simulink model "CustomLidarSLAM"  (R2024a)
settings: Solver=VariableStepAuto  StartTime=0.0  StopTime=10  RelTol=1e-3
values from neighbouring files (symbols this model uses):
  refPosesT = [180 179.9129385 179.835485475 179.767633325 179.70937525 179.660705309 179.62161846 179.592110609 179.572178633 179.56182041 179.561034833 179.569821817 ... (300 elements, 300x1)]    [refPosesT.mat]
  refPosesX = [39.2750629723 38.6655653744 38.0559809852 37.4463199178 36.8365922852 36.2268082005 35.6169777769 35.0071111275 34.3972183654 33.7873096037 33.1773949554 32.5674845338 ... (300 elements, 300x1)]    [refPosesX.mat]
  refPosesY = [28.2732997481 28.27377135 28.2751181677 28.2772382193 28.2800295229 28.2833900965 28.2872179581 28.2914111258 28.2958676177 28.3004854519 28.3051626463 28.3097972191 ... (300 elements, 300x1)]    [refPosesY.mat]
undefined symbols (not defined in the file or in its folder): Sim3dSensor
libraries: sim3dphyssensorlib x1, sim3dlib x1, sim3dautolib x1
settings Model: Creator=The MathWorks, Inc.  LastModifiedBy=FilippoOttaviani
settings SolverCC: AlgebraicLoopSolver=TrustRegion
settings DebuggingCC: UnconnectedInputMsg=warning  UnconnectedOutputMsg=warning  UnconnectedLineMsg=warning  SymbolicDimsDataTypeCodeGenerationDiagnostic=none
settings ModelReferenceCC: EnableRefExpFcnMdlSchedulingChecks=on
settings RTWCC: GPUComputeCapability=3.5  DLArmComputeVersion=19.05

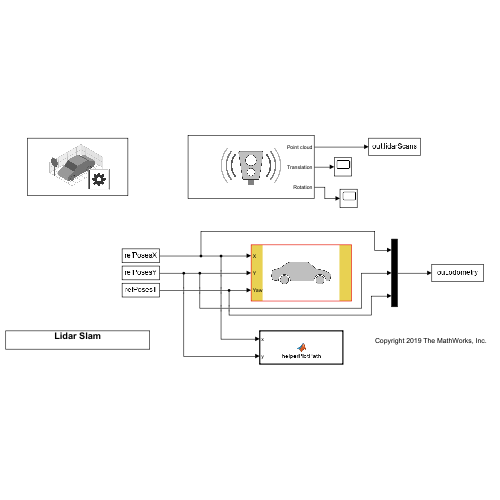
[thumbnail: Simulink's stored preview of the top-level diagram]
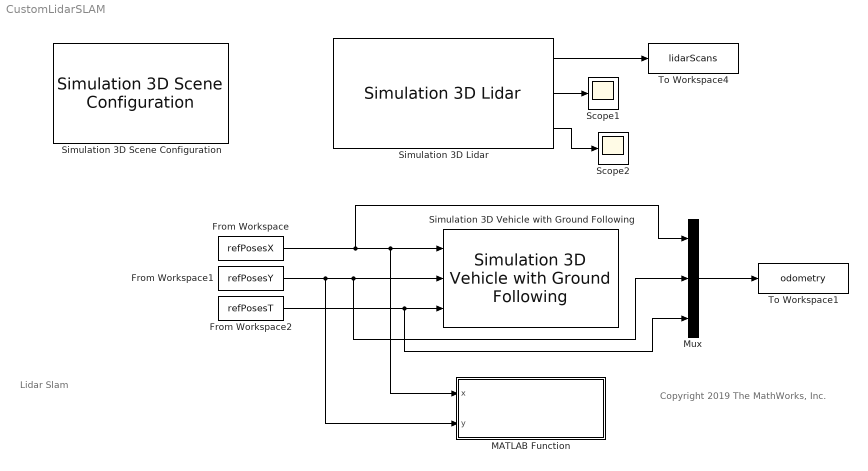
== system CustomLidarSLAM ==
  note: Copyright 2019 The MathWorks, Inc.
  note: Lidar Slam
  From Workspace : FromWorkspace  VariableName=refPosesX
  From Workspace1 : FromWorkspace  VariableName=refPosesY
  From Workspace2 : FromWorkspace  VariableName=refPosesT  Interpolate=off  OutputAfterFinalValue=Holding final value
  MATLAB Function : MATLAB Function  TreatAsAtomicUnit=on
      settings: ModelCloseFcn=|
      | % Find figure with name "Scene Display"
      | hFig = findobj('Type', 'figure', 'Name', 'Scene Display');
      | 
      | if ~isempty(hFig) && isvalid(hFig)
      |     close(hFig);
      | end
      | clear hFig;
  Mux : Mux  Inputs=3
  Scope1 : Scope
  Scope2 : Scope
  Simulation 3D Lidar : sim3dphyssensorlib/Simulation 3D Lidar  Priority=1  sensorTag=Sim3dSensor�  sensorId=1  sensorName=Sim3dSensor�  vehTagList={'Scene Origin';'SimulinkVehicle1'}  vehTag=SimulinkVehicle1  mountLoc=Roof center  offsetFlag=off  tmountOffset=[0, 0, 0]  rmountOffset=[0, 0, 0]  DetectionRange=30  RangeResolution=0.01  VerticalFOV=40  VerticalResolution=1.25  HorizontalFOV=360  HorizontalResolution=1  DistanceOutportEnabled=off  ReflectivityOutportEnabled=off  SemanticOutportEnabled=off  TransformOutportEnabled=on  SampleTime=-1  mountPoint=[-0.25 0 1.57000005245209]  mountOrientation=[0 0 0]  aMode=5  ID=1
      settings: LibrarySourceBlock=sl3dlib/Simulation 3D/Sensors/Simulation 3D Lidar
  Simulation 3D Scene Configuration : sim3dlib/Simulation 3D Scene Configuration  Priority=0  ProjectFormat=Default Scenes  SceneDesc=Large parking lot  ProjectName=C:\Program Files\MATLAB\R2024a\toolbox\shared\sim3d_projects\automotive_project_windows\UE\WindowsNoEditor\VehicleSimulation.exe  ScenePath=/Game/Maps/HwStrght  EnableOpenDRIVE=off  vehTagList={'Custom';'Scene Origin';'SimulinkVehicle1'}  vehTag=SimulinkVehicle1  FreeCameraInitialTranslation=[0, 0, 0]  FreeCameraDefaultInitialTranslation=[-6, 0, 2]  FreeCameraInitialRotation=[0, 0, 0]  FreeCameraDefaultInitialRotation=[0, -15, 0]  OpVisEn=off  Ts=1/60  EnableWindow=on  EnableRemoteAccess=off  EnableWeather=off  SunAzimuth=90  SunAltitude=40.0  EnableGeospatialSun=off  Latitude=0  Longitude=0  Date=2023-01-01  Time=10:30:00  GeoTimeZone=-5.0  SunDaylightSaving=off  wind=1  clouds=10  EnableVolumetricClouds=off  CloudCoverage=0  CloudAltitude=6  fog=0  rain=0  RaindropsEffect=off  SnowDensity=0  EnableGeospatial=off  UseTrueOrigin=off  OriginHeight=200  OriginLatitude=40.744652  OriginLongitude=-73.988864  MapStyle=Aerial  AdditionalAssetIDs=[]  UseAdvancedSunSky=off  SolarTime=11  TimeZone=-5  Day=21  Month=9  Year=2022  UseDaylightSavingTime=on  DSTStartDay=10  DSTStartMonth=3  DSTEndDay=3  DSTEndMonth=11  DSTSwitchHour=2  sensorTag=MainCamera2  sensorId=2  sensorName=MainCamera2  mountLoc=Origin  offsetFlag=off  tmountOffset=[0, 0, 0]  rmountOffset=[0, 0, 0]  HorizontalResolution=1280  VerticalResolution=720  HorizontalFOV=60  mountPoint=[0 0 0]  mountOrientation=[0 0 0]  aMode=3  ID=2  GeoTrigger=Inactive
      settings: LibrarySourceBlock=drivingsim3d/Simulation 3D Scene Configuration
  Simulation 3D Vehicle with Ground Following : sim3dautolib/Simulation 3D Vehicle with Ground Following  Priority=-1  PassVehMesh=Muscle car  MeshPath=/MathWorksSimulation/Vehicles/Muscle/Meshes/SK_MuscleCar.SK_MuscleCar  TrackWidth=1.9  WheelBase=3  WheelRadius=0.35  VehColor=Black  InitialPos=[refPosesX(1,2), refPosesY(1,2), 0]  InitialRot=[0, 0, refPosesT(1,2)]  ActorName=SimulinkVehicle1  SampleTime=-1  ActorType=SimulinkVehicle  ID=1  aMode=3  ActorTag=SimulinkVehicle1  CoordinateScheme=ISO  VehLightsControl=off  HeadlightColor=[ 1, 1, 1 ]  HighBeamIntensity=100000  LowBeamIntensity=60000  HighBeamConeAngle=70  LowBeamConeAngle=70  LeftHeadlightOrientation=[ 0, 0 ]  RightHeadlightOrientation=[ 0, 0 ]  BrakelightIntensity=500  ReverselightIntensity=500  SignallightIntensity=500  SignallightPeriod=1  SignalPulseWidth=50  TransformOutportEnabled=off
      settings: LibrarySourceBlock=drivingsim3d/Simulation 3D Vehicle with Ground Following
  To Workspace1 : ToWorkspace  VariableName=odometry  SampleTime=-1
  To Workspace4 : ToWorkspace  VariableName=lidarScans  SaveFormat=Structure With Time  SampleTime=0.1
  wires:
  From Workspace/1 -> Mux/1, Simulation 3D Vehicle with Ground Following/1, MATLAB Function/1(x)
  From Workspace1/1 -> Mux/2, Simulation 3D Vehicle with Ground Following/2, MATLAB Function/2(y)
  From Workspace2/1 -> Mux/3, Simulation 3D Vehicle with Ground Following/3
  Mux/1 -> To Workspace1/1
  Simulation 3D Lidar/2 -> Scope1/1
  Simulation 3D Lidar/3 -> Scope2/1
  Simulation 3D Lidar/1 -> To Workspace4/1

== matlab function CustomLidarSLAM/MATLAB Function ==
  settings: updateMethod=DISCRETE  sampleTime=.02
  data: x input; y input
function helperPlotPath(x, y)
%helperPlotPath Plot path on scene image
%   helperPlotPath plots the path specified by x,y waypoint on the current
%   scene.

% Copyright 2019 The MathWorks, Inc.

coder.extrinsic('helperGetCurrentScene', 'helperShowSceneImage', ...
    'figure','movegui','isvalid','images.roi.Polyline',...
    'helperUpdatePolyline');

persistent hFig hPoly;

if isempty(hFig)
    % Query the model to find the scene selection
    %sceneName = helperGetCurrentScene();
    sceneName = 'LargeParkingLot';
    
    % Create a figure and display the scene on it
    hFig = figure('Name', 'Scene Display');
    helperShowSceneImage(sceneName);
    
    % Move figure to right of screen
    movegui(hFig, 'east')
    
    % Display the path
    hold on
    hPoly = images.roi.Polyline('Parent', gca, 'Position', [x y], 'InteractionsAllowed', 'none');
end

if isvalid(hFig)
    % Update the path with the new point
    helperUpdatePolyline(hPoly, x, y);
end
end
